simulink model "Cognata_Amp_Tobi_Split_Excel"  (R2020a)
settings: Solver=VariableStepAuto  StartTime=0.0  StopTime=inf  RelTol=1e-3
model workspace (MAT data in the model file):
  WinSize = Simulink.Parameter
  WinSize.Value = 16
  WinSize.DataType = 'double'
  WinSize.Dimensions = [1 1]
  fc_bandpass = Simulink.Parameter
  fc_bandpass.Value = [0.05 0.26]
  fc_bandpass.DataType = 'double'
  fc_bandpass.Dimensions = [1 2]
undefined symbols (not defined in the file or in its folder): A1, A138674, A91496, C1, currentCFG_Cognata_Amp_Tobi_split_UB, I1, J138674, P91496, UB, W1, W91496
libraries: gtecHighspeedLib x1, gUSBamplib x1
settings Model: Creator=LAB-OREN3  LastModifiedBy=LAB-OREN3

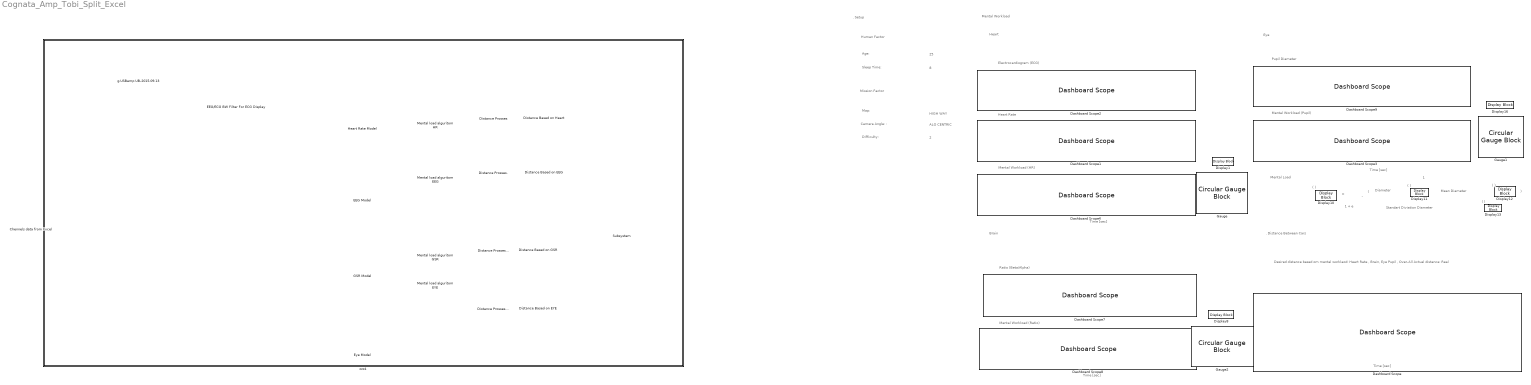
== system Cognata_Amp_Tobi_Split_Excel ==
  note: Mental Load
  note: Difficulty:
  note: Brain
  note: ( )
  note: ( )
  note: 1 + e
  note: . Setup
  note: Map:
  note: Diameter
  note: )
  note: Heart Rate
  note: Heart
  note: -
  note: ALO CENTRIC
  note: Time [sec]
  note: . Distance Between Cars
  note: Desired distance based om mental worklaod:
      | Heart Rate , Brain, Eye Pupil , Over-All
      |
      | Actual distance: Real
  note: HIGH WAY
  note: Sleep Time:
  note: 2
  note: Time [sec]
  note: Human Factor
  note: 1
  note: Electrocardiogram (ECG)
  note: Standart Diviation Diameter
  note: Mental Workload (HR)
  note: Ratio (Beta/Alpha)
  note: Time [sec]
  note: 25
  note: (
  note: 8
  note: Camera Angle: :
  note: Eye
  note: Mental Workload (Ratio)
  note: ( )
  note: =
  note: Pupil Diameter
  note: Mental Workload (Pupil)
  note: Time [sec]
  note: ( )
  note: Mission Factor
  note: Mean Diameter
  note: Mental Workload
  note: Age:
  Chennels data from Excel : Subsystem
  Dashboard Scope : DashboardScope  ShowInitialText=off  TimeSpan=10  Ymin=-1  Ymax=20  LegendPosition=Hide  ScaleAtStop=off
  Dashboard Scope1 : DashboardScope  TimeSpan=10  Ymin=0  Ymax=100  LegendPosition=Hide  ScaleAtStop=off
  Dashboard Scope2 : DashboardScope  TimeSpan=10  Ymin=-3000  Ymax=1000  LegendPosition=Hide  ScaleAtStop=off
  Dashboard Scope3 : DashboardScope  TimeSpan=10  Ymin=0  Ymax=1  LegendPosition=Hide  ScaleAtStop=off
  Dashboard Scope6 : DashboardScope  TimeSpan=10  Ymin=0  Ymax=1  LegendPosition=Hide  ScaleAtStop=off
  Dashboard Scope7 : DashboardScope  TimeSpan=10  Ymin=0  Ymax=0.5  LegendPosition=Hide  ScaleAtStop=off
  Dashboard Scope8 : DashboardScope  TimeSpan=10  Ymin=0  Ymax=1  LegendPosition=Hide  ScaleAtStop=off
  Dashboard Scope9 : DashboardScope  TimeSpan=10  Ymin=0  Ymax=5  LegendPosition=Hide  ScaleAtStop=off
  Display{1,8,10..11,13,16} (6 alike) : DisplayBlock  LabelPosition=Hide  Format=bank  Transparency=1
  Display12 : DisplayBlock  LabelPosition=Hide  Format=bank  Transparency=1  Layout=Fill available space
  Distance Based on EEG : Display
  Distance Based on EYE : Display
  Distance Based on GSR : Display
  Distance Based on Heart : Display
  Distance Prosses : MATLAB Function  TreatAsAtomicUnit=on
  Distance Prosses. : MATLAB Function  TreatAsAtomicUnit=on
  Distance Prosses... : MATLAB Function  TreatAsAtomicUnit=on
  Distance Prosses.... : MATLAB Function  TreatAsAtomicUnit=on
  EEG Model : Subsystem  ReferencedSubsystem=EEG_Ratio_Model
  EEG/ECG BW Filter For ECG Display : gtecHighspeedLib/EEG//ECG BW Filter  Order=6  LowerFreq=0.1  UpperFreq=30  SampFreq=512
      settings: SourceProductName=g.HIsys Library
  Eye Model : Subsystem  ReferencedSubsystem=Pupil_Diameter_Model
  GSR Model : Subsystem
  Gauge : CircularGaugeBlock  LabelPosition=Hide  ScaleMax=1  TickInterval=0.2
  Gauge1 : CircularGaugeBlock  LabelPosition=Hide  ScaleMax=1  TickInterval=0.2
  Gauge2 : CircularGaugeBlock  LabelPosition=Hide  ScaleMax=1  TickInterval=0.2
  Heart Rate Model : Subsystem  ReferencedSubsystem=Heart_Rate_Model
  Mental load alguritom EEG : MATLAB Function  TreatAsAtomicUnit=on
  Mental load alguritom EYE : MATLAB Function  TreatAsAtomicUnit=on
  Mental load alguritom GSR : MATLAB Function  TreatAsAtomicUnit=on
  Mental load alguritom HR : MATLAB Function  TreatAsAtomicUnit=on
  Subsystem : Subsystem
  g.USBamp UB-2015.09.13 : gUSBamplib/g.USBamp  cfg=currentCFG_Cognata_Amp_Tobi_split_UB-2015.09.13.cfg  snr=UB-2015.09.13
      settings: SourceProductName=g.USBamp
  zzz4 : Subsystem  TreatAsAtomicUnit=on
      settings: OpenFcn=% no-op
      mask Display: disp('')
  wires:
  Mental load alguritom EEG/1(y) -> Distance Prosses./1(u), Subsystem/2(Ratio)
  Distance Prosses/1(y) -> Distance Based on Heart/1
  Distance Prosses..../1(y) -> Distance Based on EYE/1
  Mental load alguritom HR/1(y) -> Distance Prosses/1(u), Subsystem/1(HR)
  Distance Prosses./1(y) -> Distance Based on EEG/1
  Mental load alguritom EYE/1(y) -> Distance Prosses..../1(u), Subsystem/4(eye)
  EEG Model/1 -> Mental load alguritom EEG/1(u)
  Eye Model/1 -> Mental load alguritom EYE/1(u)
  Heart Rate Model/2 -> Mental load alguritom HR/1(u)
  Mental load alguritom GSR/1(y) -> Distance Prosses.../1(u), Subsystem/3(GSR)
  Distance Prosses.../1(y) -> Distance Based on GSR/1
  GSR Model/1(GSR) -> Mental load alguritom GSR/1(u)
  EEG/ECG BW Filter For ECG Display/1 -> ?
  Subsystem/1(Avrage Mental Load) -> ?
  Eye Model/2 -> ?
  Eye Model/3 -> ?
  Chennels data from Excel/1(ECG) -> Heart Rate Model/1, EEG/ECG BW Filter For ECG Display/1
  Chennels data from Excel/2(EEG1) -> EEG Model/1
  Chennels data from Excel/3(EEG2) -> EEG Model/2
  Chennels data from Excel/4(EEG3) -> EEG Model/3
  Chennels data from Excel/5(EEG4) -> EEG Model/4
  Chennels data from Excel/6(EEG5) -> EEG Model/5
  Chennels data from Excel/7(EEG6) -> EEG Model/6
  Chennels data from Excel/8(EEG7) -> EEG Model/7
  Chennels data from Excel/9(EEG8) -> EEG Model/8
  Chennels data from Excel/10(EEG9) -> EEG Model/9
  Chennels data from Excel/11(EEG10) -> EEG Model/10
  Chennels data from Excel/12(EEG11) -> EEG Model/11
  Chennels data from Excel/15(Pupil diameter Left) -> Eye Model/1
  Chennels data from Excel/13(GSR) -> GSR Model/1(In1)
  Chennels data from Excel/14(Pupil diameter Right) -> Eye Model/2
  Chennels data from Excel/16(EEG12) -> EEG Model/12
  Chennels data from Excel/17(TTC) -> ?

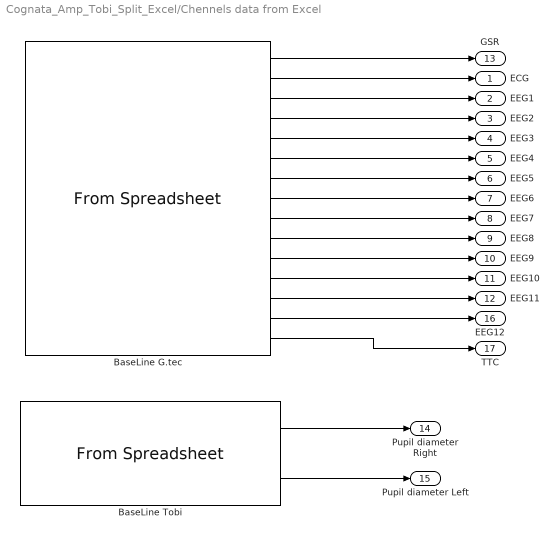
== system Cognata_Amp_Tobi_Split_Excel/Chennels data from Excel ==
  BaseLine G.tec : FromSpreadsheet  FileName=C:\Users\LAB-OREN3\Downloads\1\g.techAmp Data of A2_535986_COMBINED_CUBE_DELAY_50_TTC_15 at (15;28;36).xlsx  SheetName=גיליון1  Range=A1:A91496,C1:P91496,W1:W91496  SampleTime=0.001953125
  BaseLine Tobi : FromSpreadsheet  FileName=C:\Users\LAB-OREN3\Desktop\CognataData\Participants_DATA\Test\4\Tobii Data of A1_546053_TRAINING at (12;02;18).xlsx  SheetName=גיליון1  Range=A1:A138674,I1:J138674  SampleTime=0.001953125
  ECG : Outport
  EEG1 : Outport  Port=2
  EEG2 : Outport  Port=3
  EEG3 : Outport  Port=4
  EEG4 : Outport  Port=5
  EEG5 : Outport  Port=6
  EEG6 : Outport  Port=7
  EEG7 : Outport  Port=8
  EEG8 : Outport  Port=9
  EEG9 : Outport  Port=10
  EEG10 : Outport  Port=11
  EEG11 : Outport  Port=12
  GSR : Outport  Port=13
  Pupil diameter Right : Outport  Port=14
  Pupil diameter Left : Outport  Port=15
  EEG12 : Outport  Port=16
  TTC : Outport  Port=17
  wires:
  BaseLine G.tec/2 -> ECG/1
  BaseLine G.tec/8 -> EEG6/1
  BaseLine G.tec/13 -> EEG11/1
  BaseLine Tobi/1 -> Pupil diameter Right/1
  BaseLine G.tec/4 -> EEG2/1
  BaseLine G.tec/10 -> EEG8/1
  BaseLine G.tec/6 -> EEG4/1
  BaseLine G.tec/12 -> EEG10/1
  BaseLine G.tec/3 -> EEG1/1
  BaseLine G.tec/11 -> EEG9/1
  BaseLine G.tec/9 -> EEG7/1
  BaseLine G.tec/7 -> EEG5/1
  BaseLine G.tec/5 -> EEG3/1
  BaseLine Tobi/2 -> Pupil diameter Left/1
  BaseLine G.tec/1 -> GSR/1
  BaseLine G.tec/14 -> EEG12/1
  BaseLine G.tec/15 -> TTC/1

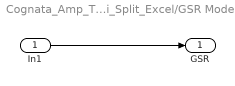
== system Cognata_Amp_Tobi_Split_Excel/GSR Model ==
  In1 : Inport
  GSR : Outport
  wires:
  In1/1 -> GSR/1

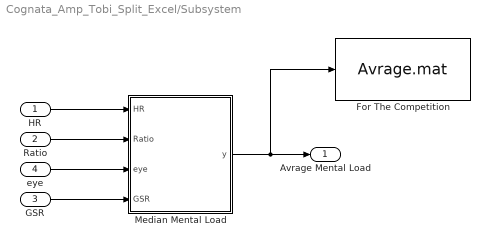
== system Cognata_Amp_Tobi_Split_Excel/Subsystem ==
  HR : Inport
  Ratio : Inport  Port=2
  GSR : Inport  Port=3
  eye : Inport  Port=4
  For The Competition : ToFile  Filename=Avrage.mat  MatrixName=Avrage
  Median Mental Load : MATLAB Function  TreatAsAtomicUnit=on
  Avrage Mental Load : Outport
  wires:
  GSR/1 -> Median Mental Load/4(GSR)
  Median Mental Load/1(y) -> For The Competition/1, Avrage Mental Load/1
  Ratio/1 -> Median Mental Load/2(Ratio)
  eye/1 -> Median Mental Load/3(eye)
  HR/1 -> Median Mental Load/1(HR)

== system Cognata_Amp_Tobi_Split_Excel/zzz4 ==

== matlab function Cognata_Amp_Tobi_Split_Excel/Distance Prosses ==
  data: u input; y output
function y = fcn(u)
%#codegen

y = (u*10)+10;

== matlab function Cognata_Amp_Tobi_Split_Excel/Mental load alguritom HR ==
  data: u input; y output
function y = fcn(u)

y= probability_of_mental_load_HR(u);

end

== matlab function Cognata_Amp_Tobi_Split_Excel/Subsystem/Median Mental Load ==
  data: HR input; y output; Ratio input; eye input; GSR input
function y = fcn(HR, Ratio, eye, GSR)


    vac = [HR Ratio,eye,GSR];
    y = median(vac);

end

== matlab function Cognata_Amp_Tobi_Split_Excel/Mental load alguritom EEG ==
  data: u input; y output
function y = fcn(u)

y= probability_of_metal_load_EEG(u);

end

== matlab function Cognata_Amp_Tobi_Split_Excel/Distance Prosses. ==
  data: u input; y output
function y = fcn(u)
%#codegen

y = (u*10)+10;

== matlab function Cognata_Amp_Tobi_Split_Excel/Mental load alguritom EYE ==
  data: u input; y output
function y = fcn( u)

y= probability_of_metal_load_EYE(u);

end

== matlab function Cognata_Amp_Tobi_Split_Excel/Distance Prosses.... ==
  data: u input; y output
function y = fcn(u)
%#codegen

y = (u*10)+10;

== matlab function Cognata_Amp_Tobi_Split_Excel/Mental load alguritom GSR ==
  data: u input; y output
function y = fcn(u)

y= probability_of_metal_load_GSR(u);

end

== matlab function Cognata_Amp_Tobi_Split_Excel/Distance Prosses... ==
  data: u input; y output
function y = fcn(u)
%#codegen

y = (u*10)+10;
